simulink model "FS_test"  (R2018a)
settings: Solver=VariableStepAuto  StartTime=0.0  StopTime=1000  RelTol=1e-3
values from neighbouring files (symbols this model uses):
  sim_speed = speed/3.6    [read_nice_I24_data.m]
  sim_time = time - time(1)    [read_nice_I24_data.m]
settings Model: Creator=Fang-Chieh Chou  LastModifiedBy=Fang-Chieh Chou

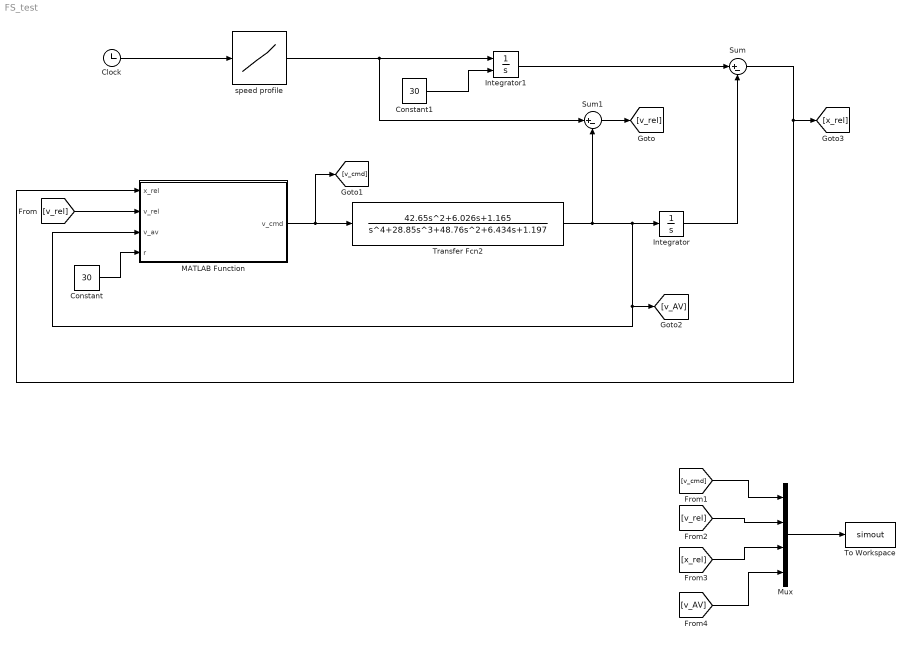
== system FS_test ==
  Clock : Clock
  Constant : Constant  Value=30
  Constant1 : Constant  Value=30
  Integrator : Integrator
  Integrator1 : Integrator  InitialConditionSource=external
  MATLAB Function : MATLAB Function  TreatAsAtomicUnit=on
  Mux : Mux
  Sum : Sum  Inputs=|+-
  Sum1 : Sum  Inputs=|+-
  To Workspace : ToWorkspace  VariableName=simout  SaveFormat=Timeseries  SampleTime=-1
  Transfer Fcn2 : TransferFcn  Numerator=[42.65 6.026 1.165]  Denominator=[1 28.85 48.76 6.434 1.197]
  speed profile : Lookup_n-D  NumberOfTableDimensions=1  BreakpointsForDimension1=sim_time  Table=sim_speed  InternalRulePriority=Speed  RndMeth=Simplest  InputSameDT=on
  wires:
  Transfer Fcn2/1 -> [v_AV], MATLAB Function/3(v_av), Integrator/1, Sum1/2
  Integrator/1 -> Sum/2
  Integrator1/1 -> Sum/1
  MATLAB Function/1(v_cmd) -> [v_cmd], Transfer Fcn2/1
  Clock/1 -> speed profile/1
  speed profile/1 -> Sum1/1, Integrator1/1
  Sum/1 -> [x_rel], MATLAB Function/1(x_rel)
  Sum1/1 -> [v_rel]
  [v_rel] -> MATLAB Function/2(v_rel)
  Constant/1 -> MATLAB Function/4(r)
  Mux/1 -> To Workspace/1
  [v_cmd] -> Mux/1
  [v_rel] -> Mux/2
  [x_rel] -> Mux/3
  [v_AV] -> Mux/4
  Constant1/1 -> Integrator1/2

== matlab function FS_test/MATLAB Function ==
  data: x_rel input; v_cmd output; v_rel input; v_av input; r input
function v_cmd = fcn(x_rel,v_rel,v_av,r)

% x_rel : relative distance (x_l - x_f)
% v_rel : relative speed  (v_l-v_f)
% v_av : subject vehicle absolute speed
% v_cmd : desired speed of the subject vehicle at next time step.
% x_rel,v_rel,v_av, and v_cmd are double arrays (matrices) of same dimension

%% follower stopper parmaeters
    w = zeros(3,1);
    alpha = zeros(3,1);
    w(1) = 4.5;
    alpha(1) = 1.5;
    w(3) = 6.0;
    alpha(3) = 0.5;
    w(2) = (w(1)+w(3))/2;
    alpha(2) = (alpha(1)+alpha(3))/2;
    if(nargin<4)
        r = 30;
    end
    
    %v_rel_star = min(v_rel,0)
    v_rel_star = v_rel;
    v_rel_star(v_rel >= 0) = 0;
   
    h_1 = 0.4;
    h_2 = 1.2;
    h_3 = 1.8;
    
    x1 = w(1) + (0.5*v_rel_star.^2)/alpha(1) + h_1*v_av;
    x2 = w(2) + (0.5*v_rel_star.^2)/alpha(2) + h_2*v_av;
    x3 = w(3) + (0.5*v_rel_star.^2)/alpha(3) + h_3*v_av;
    
    v_lead = v_av+v_rel;
    
    
    %v = min([max([v_lead,0]),r]);
    v = v_lead;
    v(v_lead<0) = 0;
    
    v(v_lead>r) = r;
  
    v_cmd = zeros(size(x_rel));  
    %safe region
    v_cmd(x_rel>x3) = r;  
    %adaptation region 1
    temp_v_cmd = v+(r-v).*(x_rel-x2)./(x3-x2);
    v_cmd(x_rel>x2 & x_rel<=x3) = temp_v_cmd(x_rel>x2 & x_rel<=x3);   
    %adaptation region 2
    temp_v_cmd = v.*(x_rel-x1)./(x2-x1);
    v_cmd(x_rel>x1 & x_rel<=x2) = temp_v_cmd(x_rel>x1 & x_rel<=x2); 
    
%     if(x_rel>x(3))
%         v_cmd = r;
%     elseif (x_rel>x(2) && x_rel<=x(3))
%         v_cmd = v*(x_rel-x(1))/(x(2)-x(1));  
%     elseif (x_rel>x(1) && x_rel <= x(2))
%         v_cmd = v+(r-v)*(x_rel-x(2))/(x(3)-x(2));
%     else
%         v_cmd = 0;
%     end
     
    
end
